simulink model "SiDLEngine"  (R2021b)
settings: Solver=VariableStepAuto  StartTime=0.0  StopTime=inf  FixedStep=0.03  RelTol=1e-3  EnableMultiTasking=on
model workspace (MAT data in the model file):
  AfrStoich = Simulink.Parameter
  AfrStoich.Value = 14.6
  AfrStoich.DataType = 'double'
  AfrStoich.Complexity = 'real'
  AfrStoich.Dimensions = [1 1]
  Cps = Simulink.Parameter
  Cps.Value = 2
  Cps.DataType = 'double'
  Cps.Complexity = 'real'
  Cps.Dimensions = [1 1]
  FuelSg = Simulink.Parameter
  FuelSg.Value = 0.75
  FuelSg.DataType = 'double'
  FuelSg.Complexity = 'real'
  FuelSg.Dimensions = [1 1]
  NCyl = Simulink.Parameter
  NCyl.Value = 4
  NCyl.DataType = 'double'
  NCyl.Complexity = 'real'
  NCyl.Dimensions = [1 1]
  Pstd = Simulink.Parameter
  Pstd.Value = 101325
  Pstd.DataType = 'double'
  Pstd.Complexity = 'real'
  Pstd.Dimensions = [1 1]
  Rair = Simulink.Parameter
  Rair.Value = 287
  Rair.DataType = 'double'
  Rair.Complexity = 'real'
  Rair.Dimensions = [1 1]
  TimeCnstECP = Simulink.Parameter
  TimeCnstECP.Value = 0.01
  TimeCnstECP.DataType = 'double'
  TimeCnstECP.Complexity = 'real'
  TimeCnstECP.Dimensions = [1 1]
  TimeCnstEGR = Simulink.Parameter
  TimeCnstEGR.Value = 0.01
  TimeCnstEGR.DataType = 'double'
  TimeCnstEGR.Complexity = 'real'
  TimeCnstEGR.Dimensions = [1 1]
  TimeCnstETC = Simulink.Parameter
  TimeCnstETC.Value = 0.01
  TimeCnstETC.DataType = 'double'
  TimeCnstETC.Complexity = 'real'
  TimeCnstETC.Dimensions = [1 1]
  TimeCnstICP = Simulink.Parameter
  TimeCnstICP.Value = 0.01
  TimeCnstICP.DataType = 'double'
  TimeCnstICP.Complexity = 'real'
  TimeCnstICP.Dimensions = [1 1]
  TimeCnstIVL = Simulink.Parameter
  TimeCnstIVL.Value = 0.125
  TimeCnstIVL.DataType = 'double'
  TimeCnstIVL.Complexity = 'real'
  TimeCnstIVL.Dimensions = [1 1]
  TimeCnstMFA = Simulink.Parameter
  TimeCnstMFA.Value = 0.125
  TimeCnstMFA.DataType = 'double'
  TimeCnstMFA.Complexity = 'real'
  TimeCnstMFA.Dimensions = [1 1]
  TimeCnstSWVA = Simulink.Parameter
  TimeCnstSWVA.Value = 0.125
  TimeCnstSWVA.DataType = 'double'
  TimeCnstSWVA.Complexity = 'real'
  TimeCnstSWVA.Dimensions = [1 1]
  TimeCnstVCR = Simulink.Parameter
  TimeCnstVCR.Value = 0.125
  TimeCnstVCR.DataType = 'double'
  TimeCnstVCR.Complexity = 'real'
  TimeCnstVCR.Dimensions = [1 1]
  TimeCnstVGT = Simulink.Parameter
  TimeCnstVGT.Value = 0.15
  TimeCnstVGT.DataType = 'double'
  TimeCnstVGT.Complexity = 'real'
  TimeCnstVGT.Dimensions = [1 1]
  TimeCnstVIRL = Simulink.Parameter
  TimeCnstVIRL.Value = 0.125
  TimeCnstVIRL.DataType = 'double'
  TimeCnstVIRL.Complexity = 'real'
  TimeCnstVIRL.Dimensions = [1 1]
  TimeCnstWGA = Simulink.Parameter
  TimeCnstWGA.Value = 0.01
  TimeCnstWGA.DataType = 'double'
  TimeCnstWGA.Complexity = 'real'
  TimeCnstWGA.Dimensions = [1 1]
  Ts = Simulink.Parameter
  Ts.Value = 0.01
  Ts.DataType = 'double'
  Ts.Complexity = 'real'
  Ts.Dimensions = [1 1]
  Tstd = Simulink.Parameter
  Tstd.Value = 293.15
  Tstd.DataType = 'double'
  Tstd.Complexity = 'real'
  Tstd.Dimensions = [1 1]
  Vd = Simulink.Parameter
  Vd.Value = 0.0015
  Vd.DataType = 'double'
  Vd.Complexity = 'real'
  Vd.Dimensions = [1 1]
  layer2Bias = Simulink.Parameter
  layer2Bias.Value = [-0.102818198502 -0.0669189542532 -0.0175336152315 -0.0613032355905 -0.0570961982012 -0.061625469476 -0.0630445405841 -0.102546460927 -0.0423759259284 -0.0306564457715 -0.0652378797531 -0.129787817597 ... (800 elements, 800x1)]
  layer2Bias.DataType = 'single'
  layer2Bias.Complexity = 'real'
  layer2Bias.Dimensions = [800 1]
  layer2InputWeights = Simulink.Parameter
  layer2InputWeights.Value = [-0.0867959260941 0.0265881456435 -0.00261938013136 0.0648385435343 -0.0334306880832 -0.044301789254 0.0604524612427 0.00893297791481 -0.0994751527905 0.0255589019507 -0.122370123863 -0.0740034654737 ... (1600 elements, 800x2)]
  layer2InputWeights.DataType = 'single'
  layer2InputWeights.Complexity = 'real'
  layer2InputWeights.Dimensions = [800 2]
  layer2RecurrentWeights = Simulink.Parameter
  layer2RecurrentWeights.Value = [-0.015235141851 -0.11403311789 0.112884886563 0.0588350631297 0.0682250186801 0.0444636531174 -0.0968889594078 -0.0397337339818 -0.0227067749947 0.0294026453048 -0.0304179247469 -0.145884677768 ... (160000 elements, 800x200)]
  layer2RecurrentWeights.DataType = 'single'
  layer2RecurrentWeights.Complexity = 'real'
  layer2RecurrentWeights.Dimensions = [800 200]
  layer3Bias = Simulink.Parameter
  layer3Bias.Value = [0.0529259070754; 0.0636636316776; 0.0140457563102; 0.0780845806003; 0.0347621031106; -0.023198319599; -0.0368600413203; -0.00711429771036; -0.0257519558072; 0.0254531633109; 0.0144603000954]
  layer3Bias.DataType = 'single'
  layer3Bias.Complexity = 'real'
  layer3Bias.Dimensions = [11 1]
  layer3Weights = Simulink.Parameter
  layer3Weights.Value = [0.0566984564066 0.0242331400514 0.158808469772 0.0399505831301 -0.0030719502829 0.0837587192655 0.0579013302922 -0.0333247296512 -0.120384372771 -0.125806882977 0.0938690528274 -0.052338026464 ... (2200 elements, 11x200)]
  layer3Weights.DataType = 'single'
  layer3Weights.Complexity = 'real'
  layer3Weights.Dimensions = [11 200]
  muX = Simulink.Parameter
  muX.Value = [2220.83734119 107.92815484]
  muX.DataType = 'double'
  muX.Complexity = 'real'
  muX.Dimensions = [1 2]
  muY = Simulink.Parameter
  muY.Value = [104.671657967 115562.072489 0.00224719893222 986.056400633 7383.06398882 0.0299760704621 325.741103054 5.88867806863e-05 0.000942478781448 3.56158507349e-05 0.00543639293543]
  muY.DataType = 'double'
  muY.Complexity = 'real'
  muY.Dimensions = [1 11]
  sigX = Simulink.Parameter
  sigX.Value = [1470.27383875 63.5647381428]
  sigX.DataType = 'double'
  sigX.Complexity = 'real'
  sigX.Dimensions = [1 2]
  sigY = Simulink.Parameter
  sigY.Value = [65.6275263528 46686.4071583 0.00207427504126 224.539922164 5111.0011239 0.0252132241042 8.06209455442 0.000125926264941 0.00171123843744 4.89959895827e-05 0.00480295587248]
  sigY.DataType = 'double'
  sigY.Complexity = 'real'
  sigY.Dimensions = [1 11]
libraries: autolibutils x4, simulink x2, autolibsharedmappedenginescommon x1, autolibpowerinfoutils x1
settings Model: DataDictionary=SiDLEngine.sldd  ModifiedByFormat=The MathWorks, Inc.  Creator=The MathWorks, Inc.  LastModifiedBy=The MathWorks, Inc.
settings SolverCC: AlgebraicLoopSolver=TrustRegion  DecoupledContinuousIntegration=on
settings DataIOCC: DSMLogging=off  ReturnWorkspaceOutputs=off
settings DebuggingCC: SFMachineParentedDataDiag=warning  ArithmeticOperatorsInVariantConditions=warning
settings SFSimCC: SimUseLocalCustomCode=off
settings RTWCC: RTWUseLocalCustomCode=off
settings CodeAppCC: StateflowObjectComments=on
settings GRTTargetCC: TargetLangStandard=C89/C90 (ANSI)
settings ConfigComp: CovMetricSettings=dsw  CovSaveCumulativeToWorkspaceVar=on  CovSaveSingleToWorkspaceVar=on  CovExternalEMLEnable=off
settings SimscapeCC: SimscapeNormalizeSystem=off  SimscapeNominalValues={1, 'bar'; 1, 'cm^3/s'; 1, 'bar*kg/s'; 1, 'kJ/kg'; 1, 'kW'}

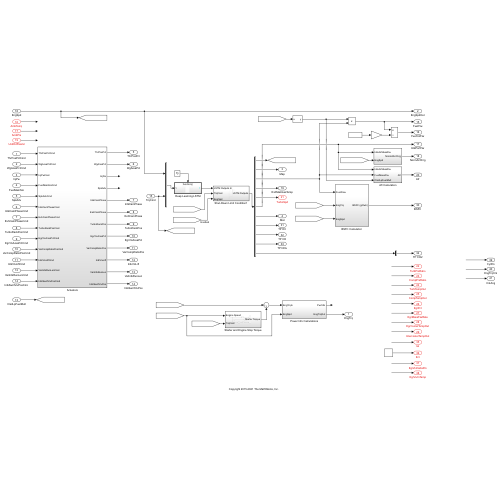
[thumbnail: Simulink's stored preview of the top-level diagram]
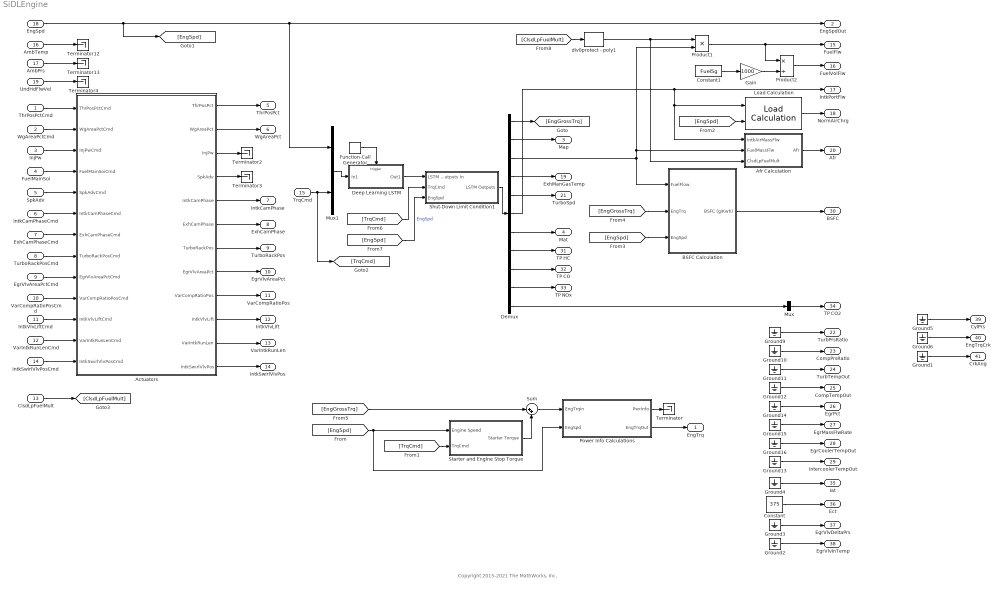
== system SiDLEngine ==
  note: Copyright 2015-2021 The MathWorks, Inc.
  ThrPosPctCmd : Inport
  WgAreaPctCmd : Inport  Port=2
  InjPw : Inport  Port=3
  FuelMainSoi : Inport  Port=4
  SpkAdv : Inport  Port=5
  IntkCamPhaseCmd : Inport  Port=6
  ExhCamPhaseCmd : Inport  Port=7
  TurboRackPosCmd : Inport  Port=8
  EgrVlvAreaPctCmd : Inport  Port=9
  VarCompRatioPosCmd : Inport  Port=10
  IntkVlvLiftCmd : Inport  Port=11
  VarIntkRunLenCmd : Inport  Port=12
  ClsdLpFuelMult : Inport  Port=13  Unit=1
  IntkSwirlVlvPosCmd : Inport  Port=14
  TrqCmd : Inport  Port=15  Unit=N*m
  AmbTemp : Inport  Port=16  Unit=K
  AmbPrs : Inport  Port=17  Unit=Pa
  EngSpd : Inport  Port=18  Interpolate=off
  UndHdFlwVel : Inport  Port=19  Unit=m/s
  Actuators : Subsystem
  Afr Calculation : Subsystem
  BSFC Calculation : Subsystem
  Constant : Constant  Value=375
  Constant1 : Constant  Value=FuelSg
  Deep Learning LSTM : Subsystem  TreatAsAtomicUnit=on
  Demux : Demux  Outputs=11
  Function-Call Generator : simulink/Ports & Subsystems/Function-Call Generator  sample_time=Ts  numberOfIterations=1  DisallowWideOutput=off
  Gain : Gain  Gain=1000
  Ground{1..6,9..16} (14 alike) : Ground
  Load Calculation : autolibsharedmappedenginescommon/Load Calculation  SystemSampleTime=-1  VariantActivationTime=update diagram  Latency=0  AutoFrameSizeCalculation=off
      settings: SourceProductBaseCode=PW,DR,MT,UV,VE
  Mux : Mux  Inputs=1
  Mux1 : Mux  Inputs=2
  Power Info Calculations : Subsystem
  Product1 : Product
  Product2 : Product  Inputs=*/
  Shut-Down Limit Condition1 : Subsystem
  Starter and Engine Stop Torque : Subsystem
  Sum : Sum  Inputs=|++
  Terminator{,2..4,12..13} (6 alike) : Terminator
  div0protect - poly1 : autolibutils/div0protect - poly  thresh=0.01  ZeroCross1=off  aMode=aMode
      settings: SourceProductBaseCode=PW,DR,MT,UV,VE
  EngTrq : Outport  Unit=N*m  VectorParamsAs1DForOutWhenUnconnected=off
  EngSpdOut : Outport  Port=2  VectorParamsAs1DForOutWhenUnconnected=off
  Map : Outport  Port=3  Unit=Pa  VectorParamsAs1DForOutWhenUnconnected=off
  Mat : Outport  Port=4  Unit=K  VectorParamsAs1DForOutWhenUnconnected=off
  ThrPosPct : Outport  Port=5  VectorParamsAs1DForOutWhenUnconnected=off
  WgAreaPct : Outport  Port=6  VectorParamsAs1DForOutWhenUnconnected=off
  IntkCamPhase : Outport  Port=7  VectorParamsAs1DForOutWhenUnconnected=off
  ExhCamPhase : Outport  Port=8  VectorParamsAs1DForOutWhenUnconnected=off
  TurboRackPos : Outport  Port=9  VectorParamsAs1DForOutWhenUnconnected=off
  EgrVlvAreaPct : Outport  Port=10  VectorParamsAs1DForOutWhenUnconnected=off
  VarCompRatioPos : Outport  Port=11  VectorParamsAs1DForOutWhenUnconnected=off
  IntkVlvLift : Outport  Port=12  VectorParamsAs1DForOutWhenUnconnected=off
  VarIntkRunLen : Outport  Port=13  VectorParamsAs1DForOutWhenUnconnected=off
  IntkSwirlVlvPos : Outport  Port=14  VectorParamsAs1DForOutWhenUnconnected=off
  FuelFlw : Outport  Port=15  Unit=kg/s  VectorParamsAs1DForOutWhenUnconnected=off
  FuelVolFlw : Outport  Port=16  Unit=m^3/s  VectorParamsAs1DForOutWhenUnconnected=off
  IntkPortFlw : Outport  Port=17  Unit=kg/s  VectorParamsAs1DForOutWhenUnconnected=off
  NormAirChrg : Outport  Port=18  Unit=1  VectorParamsAs1DForOutWhenUnconnected=off
  ExhManGasTemp : Outport  Port=19  Unit=K  VectorParamsAs1DForOutWhenUnconnected=off
  Afr : Outport  Port=20  Unit=1  VectorParamsAs1DForOutWhenUnconnected=off
  TurboSpd : Outport  Port=21  Unit=rad/s  VectorParamsAs1DForOutWhenUnconnected=off
  TurbPrsRatio : Outport  Port=22  Unit=1  VectorParamsAs1DForOutWhenUnconnected=off
  CompPrsRatio : Outport  Port=23  Unit=1  VectorParamsAs1DForOutWhenUnconnected=off
  TurbTempOut : Outport  Port=24  Unit=K  VectorParamsAs1DForOutWhenUnconnected=off
  CompTempOut : Outport  Port=25  Unit=K  VectorParamsAs1DForOutWhenUnconnected=off
  EgrPct : Outport  Port=26  Unit=%  VectorParamsAs1DForOutWhenUnconnected=off
  EgrMassFlwRate : Outport  Port=27  Unit=kg/s  VectorParamsAs1DForOutWhenUnconnected=off
  EgrCoolerTempOut : Outport  Port=28  Unit=K  VectorParamsAs1DForOutWhenUnconnected=off
  IntercoolerTempOut : Outport  Port=29  Unit=K  VectorParamsAs1DForOutWhenUnconnected=off
  BSFC : Outport  Port=30  Unit=g/(kW*hr)  VectorParamsAs1DForOutWhenUnconnected=off
  TP HC : Outport  Port=31  Unit=kg/s  VectorParamsAs1DForOutWhenUnconnected=off
  TP CO : Outport  Port=32  Unit=kg/s  VectorParamsAs1DForOutWhenUnconnected=off
  TP NOx : Outport  Port=33  Unit=kg/s  VectorParamsAs1DForOutWhenUnconnected=off
  TP CO2 : Outport  Port=34  Unit=kg/s  VectorParamsAs1DForOutWhenUnconnected=off
  Iat : Outport  Port=35  Unit=K  VectorParamsAs1DForOutWhenUnconnected=off
  Ect : Outport  Port=36  Unit=K  VectorParamsAs1DForOutWhenUnconnected=off
  EgrVlvDeltaPrs : Outport  Port=37  Unit=Pa  VectorParamsAs1DForOutWhenUnconnected=off
  EgrVlvInTemp : Outport  Port=38  Unit=K  VectorParamsAs1DForOutWhenUnconnected=off
  CylPrs : Outport  Port=39  VectorParamsAs1DForOutWhenUnconnected=off
  EngTrqCrk : Outport  Port=40  VectorParamsAs1DForOutWhenUnconnected=off
  CrkAng : Outport  Port=41  VectorParamsAs1DForOutWhenUnconnected=off
  wires:
  Demux/6 -> Load Calculation/1, Afr Calculation/1(IntkAirMassFlw), IntkPortFlw/1
  Demux/11 -> Mux/1
  Demux/9 -> TP CO/1
  Mux/1 -> TP CO2/1
  IntkCamPhaseCmd/1 -> Actuators/6(IntkCamPhaseCmd)
  Ground16/1 -> EgrCoolerTempOut/1
  Ground13/1 -> IntercoolerTempOut/1
  Ground12/1 -> CompTempOut/1
  FuelMainSoi/1 -> Actuators/4(FuelMainSoiCmd)
  EgrVlvAreaPctCmd/1 -> Actuators/9(EgrVlvAreaPctCmd)
  Ground11/1 -> TurbTempOut/1
  ExhCamPhaseCmd/1 -> Actuators/7(ExhCamPhaseCmd)
  Ground9/1 -> TurbPrsRatio/1
  SpkAdv/1 -> Actuators/5(SpkAdvCmd)
  AmbTemp/1 -> Terminator12/1
  Ground15/1 -> EgrMassFlwRate/1
  TurboRackPosCmd/1 -> Actuators/8(TurboRackPosCmd)
  ThrPosPctCmd/1 -> Actuators/1(ThrPosPctCmd)
  WgAreaPctCmd/1 -> Actuators/2(WgAreaPctCmd)
  InjPw/1 -> Actuators/3(InjPwCmd)
  Ground10/1 -> CompPrsRatio/1
  Demux/7 -> Mat/1
  Demux/2 -> Map/1
  AmbPrs/1 -> Terminator13/1
  IntkVlvLiftCmd/1 -> Actuators/11(IntkVlvLiftCmd)
  VarCompRatioPosCmd/1 -> Actuators/10(VarCompRatioPosCmd)
  VarIntkRunLenCmd/1 -> Actuators/12(VarIntkRunLenCmd)
  IntkSwirlVlvPosCmd/1 -> Actuators/13(IntkSwirlVlvPosCmd)
  UndHdFlwVel/1 -> Terminator4/1
  Actuators/5(IntkCamPhase) -> IntkCamPhase/1
  Actuators/6(ExhCamPhase) -> ExhCamPhase/1
  Actuators/7(TurboRackPos) -> TurboRackPos/1
  Actuators/8(EgrVlvAreaPct) -> EgrVlvAreaPct/1
  Actuators/9(VarCompRatioPos) -> VarCompRatioPos/1
  Actuators/10(IntkVlvLift) -> IntkVlvLift/1
  Actuators/11(VarIntkRunLen) -> VarIntkRunLen/1
  Actuators/12(IntkSwirlVlvPos) -> IntkSwirlVlvPos/1
  Constant/1 -> Ect/1
  Ground2/1 -> EgrVlvInTemp/1
  Ground3/1 -> EgrVlvDeltaPrs/1
  Ground4/1 -> Iat/1
  Power Info Calculations/1(PwrInfo) -> Terminator/1
  Demux/3 -> Afr Calculation/2(FuelMassFlw), Product1/2, BSFC Calculation/1(FuelFlow)
  Product2/1 -> FuelVolFlw/1
  ClsdLpFuelMult/1 -> [ClsdLpFuelMult]
  Deep Learning LSTM/1(Out1) -> Shut-Down Limit Condition1/1(LSTM Outputs In)
  Demux/4 -> ExhManGasTemp/1
  Demux/5 -> TurboSpd/1
  Constant1/1 -> Gain/1
  Starter and Engine Stop Torque/1(Starter Torque) -> Sum/2
  Sum/1 -> Power Info Calculations/1(EngTrqIn)
  Function-Call Generator/1 -> Deep Learning LSTM/Trigger
  Ground14/1 -> EgrPct/1
  Gain/1 -> Product2/2
  Power Info Calculations/2(EngTrqOut) -> EngTrq/1
  [EngSpd] -> Starter and Engine Stop Torque/1(Engine Speed), Power Info Calculations/2(EngSpd)
  Afr Calculation/1(Afr) -> Afr/1
  Load Calculation/1 -> NormAirChrg/1
  [EngSpd] -> Load Calculation/2
  BSFC Calculation/1(BSFC (g/Kwh)) -> BSFC/1
  [EngSpd] -> BSFC Calculation/3(EngSpd)
  [EngGrossTrq] -> BSFC Calculation/2(EngTrq)
  [TrqCmd] -> Starter and Engine Stop Torque/2(TrqCmd)
  Shut-Down Limit Condition1/1(LSTM Outputs) -> Demux/1
  [EngSpd] -> Shut-Down Limit Condition1/3(EngSpd)  "EngSpd"
  EngSpd/1 -> [EngSpd], Mux1/1, EngSpdOut/1
  Actuators/1(ThrPosPct) -> ThrPosPct/1
  Actuators/2(WgAreaPct) -> WgAreaPct/1
  Actuators/3(InjPw) -> Terminator2/1
  Actuators/4(SpkAdv) -> Terminator3/1
  [EngGrossTrq] -> Sum/1
  Mux1/1 -> Deep Learning LSTM/1(In1)
  Demux/1 -> [EngGrossTrq]
  TrqCmd/1 -> [TrqCmd], Mux1/2
  Demux/8 -> TP HC/1
  Demux/10 -> TP NOx/1
  [TrqCmd] -> Shut-Down Limit Condition1/2(TrqCmd)
  [ClsdLpFuelMult] -> div0protect - poly1/1
  Product1/1 -> Product2/1, FuelFlw/1
  div0protect - poly1/1 -> Afr Calculation/3(ClsdLpFuelMult), Product1/1
  Ground5/1 -> CylPrs/1
  Ground6/1 -> EngTrqCrk/1
  Ground1/1 -> CrkAng/1

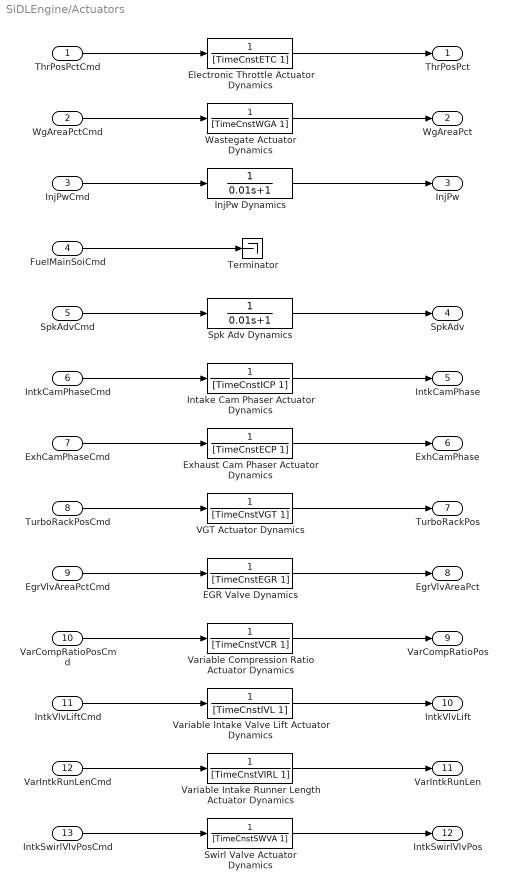
== system SiDLEngine/Actuators ==
  ThrPosPctCmd : Inport  Unit=%
  WgAreaPctCmd : Inport  Port=2  Unit=%
  InjPwCmd : Inport  Port=3  Unit=ms
  FuelMainSoiCmd : Inport  Port=4  Unit=deg
  SpkAdvCmd : Inport  Port=5  Unit=deg
  IntkCamPhaseCmd : Inport  Port=6  Unit=deg
  ExhCamPhaseCmd : Inport  Port=7  Unit=deg
  TurboRackPosCmd : Inport  Port=8  Unit=1
  EgrVlvAreaPctCmd : Inport  Port=9  Unit=%
  VarCompRatioPosCmd : Inport  Port=10
  IntkVlvLiftCmd : Inport  Port=11
  VarIntkRunLenCmd : Inport  Port=12
  IntkSwirlVlvPosCmd : Inport  Port=13
  EGR Valve Dynamics : TransferFcn  Denominator=[TimeCnstEGR 1]
  Electronic Throttle Actuator Dynamics : TransferFcn  Denominator=[TimeCnstETC 1]
  Exhaust Cam Phaser Actuator Dynamics : TransferFcn  Denominator=[TimeCnstECP 1]
  InjPw Dynamics : TransferFcn  Denominator=[0.01 1]
  Intake Cam Phaser Actuator Dynamics : TransferFcn  Denominator=[TimeCnstICP 1]
  Spk Adv Dynamics : TransferFcn  Denominator=[0.01 1]
  Swirl Valve Actuator Dynamics : TransferFcn  Denominator=[TimeCnstSWVA 1]
  Terminator : Terminator
  VGT Actuator Dynamics : TransferFcn  Denominator=[TimeCnstVGT 1]
  Variable Compression Ratio Actuator Dynamics : TransferFcn  Denominator=[TimeCnstVCR 1]
  Variable Intake Runner Length Actuator Dynamics : TransferFcn  Denominator=[TimeCnstVIRL 1]
  Variable Intake Valve Lift Actuator Dynamics : TransferFcn  Denominator=[TimeCnstIVL 1]
  Wastegate Actuator Dynamics : TransferFcn  Denominator=[TimeCnstWGA 1]
  ThrPosPct : Outport  Unit=%  VectorParamsAs1DForOutWhenUnconnected=off
  WgAreaPct : Outport  Port=2  Unit=%  VectorParamsAs1DForOutWhenUnconnected=off
  InjPw : Outport  Port=3  VectorParamsAs1DForOutWhenUnconnected=off
  SpkAdv : Outport  Port=4  VectorParamsAs1DForOutWhenUnconnected=off
  IntkCamPhase : Outport  Port=5  Unit=deg  VectorParamsAs1DForOutWhenUnconnected=off
  ExhCamPhase : Outport  Port=6  Unit=deg  VectorParamsAs1DForOutWhenUnconnected=off
  TurboRackPos : Outport  Port=7  Unit=1  VectorParamsAs1DForOutWhenUnconnected=off
  EgrVlvAreaPct : Outport  Port=8  Unit=%  VectorParamsAs1DForOutWhenUnconnected=off
  VarCompRatioPos : Outport  Port=9  VectorParamsAs1DForOutWhenUnconnected=off
  IntkVlvLift : Outport  Port=10  VectorParamsAs1DForOutWhenUnconnected=off
  VarIntkRunLen : Outport  Port=11  VectorParamsAs1DForOutWhenUnconnected=off
  IntkSwirlVlvPos : Outport  Port=12  VectorParamsAs1DForOutWhenUnconnected=off
  wires:
  Variable Compression Ratio Actuator Dynamics/1 -> VarCompRatioPos/1
  Variable Intake Valve Lift Actuator Dynamics/1 -> IntkVlvLift/1
  Variable Intake Runner Length Actuator Dynamics/1 -> VarIntkRunLen/1
  Swirl Valve Actuator Dynamics/1 -> IntkSwirlVlvPos/1
  Intake Cam Phaser Actuator Dynamics/1 -> IntkCamPhase/1
  Exhaust Cam Phaser Actuator Dynamics/1 -> ExhCamPhase/1
  Wastegate Actuator Dynamics/1 -> WgAreaPct/1
  Electronic Throttle Actuator Dynamics/1 -> ThrPosPct/1
  FuelMainSoiCmd/1 -> Terminator/1
  IntkVlvLiftCmd/1 -> Variable Intake Valve Lift Actuator Dynamics/1
  IntkSwirlVlvPosCmd/1 -> Swirl Valve Actuator Dynamics/1
  WgAreaPctCmd/1 -> Wastegate Actuator Dynamics/1
  ThrPosPctCmd/1 -> Electronic Throttle Actuator Dynamics/1
  ExhCamPhaseCmd/1 -> Exhaust Cam Phaser Actuator Dynamics/1
  IntkCamPhaseCmd/1 -> Intake Cam Phaser Actuator Dynamics/1
  VarCompRatioPosCmd/1 -> Variable Compression Ratio Actuator Dynamics/1
  VarIntkRunLenCmd/1 -> Variable Intake Runner Length Actuator Dynamics/1
  InjPwCmd/1 -> InjPw Dynamics/1
  VGT Actuator Dynamics/1 -> TurboRackPos/1
  EGR Valve Dynamics/1 -> EgrVlvAreaPct/1
  TurboRackPosCmd/1 -> VGT Actuator Dynamics/1
  EgrVlvAreaPctCmd/1 -> EGR Valve Dynamics/1
  SpkAdvCmd/1 -> Spk Adv Dynamics/1
  Spk Adv Dynamics/1 -> SpkAdv/1
  InjPw Dynamics/1 -> InjPw/1

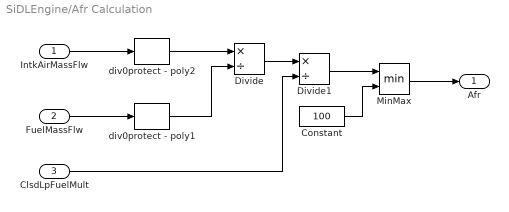
== system SiDLEngine/Afr Calculation ==
  IntkAirMassFlw : Inport  Unit=kg/s
  FuelMassFlw : Inport  Port=2  Unit=kg/s
  ClsdLpFuelMult : Inport  Port=3  Unit=kg/s
  Constant : Constant  Value=100
  Divide : Product  Inputs=*/
  Divide1 : Product  Inputs=*/
  MinMax : MinMax  Inputs=2  ZeroCross=off
  div0protect - poly1 : autolibutils/div0protect - poly  thresh=1e-9  ZeroCross1=off  aMode=aMode
      settings: SourceProductBaseCode=PW,DR,MT,UV,VE
  div0protect - poly2 : autolibutils/div0protect - poly  thresh=100e-9  ZeroCross1=off  aMode=aMode
      settings: SourceProductBaseCode=PW,DR,MT,UV,VE
  Afr : Outport  Unit=1  VectorParamsAs1DForOutWhenUnconnected=off
  wires:
  MinMax/1 -> Afr/1
  div0protect - poly1/1 -> Divide/2
  Divide/1 -> Divide1/1
  div0protect - poly2/1 -> Divide/1
  Constant/1 -> MinMax/2
  IntkAirMassFlw/1 -> div0protect - poly2/1
  FuelMassFlw/1 -> div0protect - poly1/1
  ClsdLpFuelMult/1 -> Divide1/2
  Divide1/1 -> MinMax/1

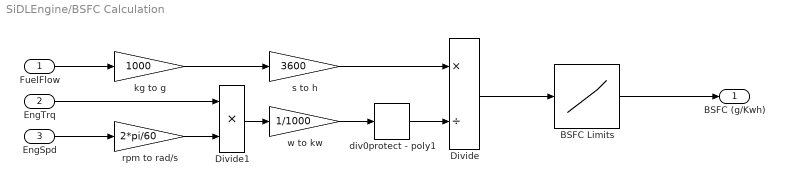
== system SiDLEngine/BSFC Calculation ==
  FuelFlow : Inport
  EngTrq : Inport  Port=2
  EngSpd : Inport  Port=3
  BSFC Limits : Lookup_n-D  NumberOfTableDimensions=1  BreakpointsForDimension1=[0 500]  Table=[0 500]  ExtrapMethod=Clip  InternalRulePriority=Speed  RndMeth=Simplest  InputSameDT=on
  Divide : Product  Inputs=*/
  Divide1 : Product  Inputs=**
  div0protect - poly1 : autolibutils/div0protect - poly  thresh=1e-6  ZeroCross1=off  aMode=aMode
      settings: SourceProductBaseCode=PW,DR,MT,UV,VE
  kg to g : Gain  Gain=1000
  rpm to rad/s : Gain  Gain=2*pi/60
  s to h : Gain  Gain=3600
  w to kw : Gain  Gain=1/1000
  BSFC (g/Kwh) : Outport  VectorParamsAs1DForOutWhenUnconnected=off
  wires:
  Divide1/1 -> w to kw/1
  kg to g/1 -> s to h/1
  FuelFlow/1 -> kg to g/1
  rpm to rad/s/1 -> Divide1/2
  EngSpd/1 -> rpm to rad/s/1
  EngTrq/1 -> Divide1/1
  Divide/1 -> BSFC Limits/1
  w to kw/1 -> div0protect - poly1/1
  s to h/1 -> Divide/1
  BSFC Limits/1 -> BSFC (g/Kwh)/1
  div0protect - poly1/1 -> Divide/2

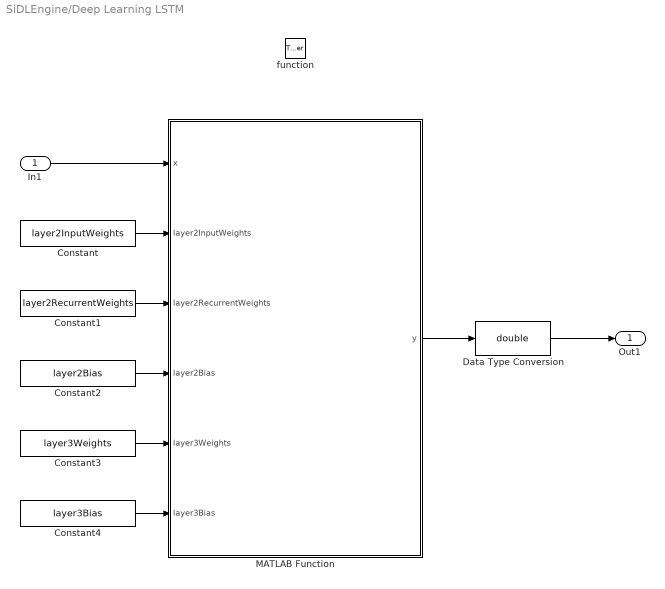
== system SiDLEngine/Deep Learning LSTM ==
  In1 : Inport
  function : TriggerPort  TriggerType=function-call  VariantControl=Variant
  Constant : Constant  Value=layer2InputWeights
  Constant1 : Constant  Value=layer2RecurrentWeights
  Constant2 : Constant  Value=layer2Bias
  Constant3 : Constant  Value=layer3Weights
  Constant4 : Constant  Value=layer3Bias
  Data Type Conversion : DataTypeConversion  OutDataTypeStr=double
  MATLAB Function : MATLAB Function  TreatAsAtomicUnit=on
  Out1 : Outport  VectorParamsAs1DForOutWhenUnconnected=off
  wires:
  In1/1 -> MATLAB Function/1(x)
  MATLAB Function/1(y) -> Data Type Conversion/1
  Data Type Conversion/1 -> Out1/1
  Constant/1 -> MATLAB Function/2(layer2InputWeights)
  Constant1/1 -> MATLAB Function/3(layer2RecurrentWeights)
  Constant2/1 -> MATLAB Function/4(layer2Bias)
  Constant3/1 -> MATLAB Function/5(layer3Weights)
  Constant4/1 -> MATLAB Function/6(layer3Bias)

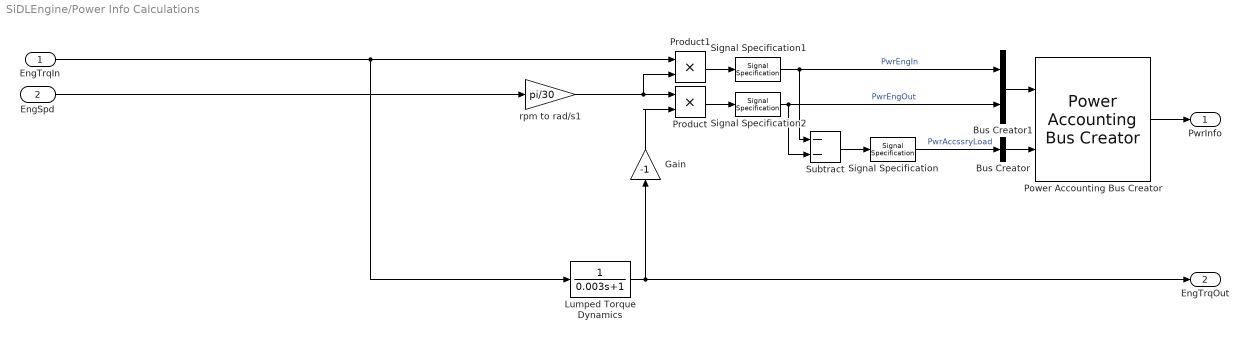
== system SiDLEngine/Power Info Calculations ==
  EngTrqIn : Inport
  EngSpd : Inport  Port=2
  Bus Creator : BusCreator  Inputs=1
  Bus Creator1 : BusCreator  Inputs=2
  Gain : Gain  Gain=-1
  Lumped Torque Dynamics : TransferFcn  Denominator=[0.003 1]
  Power Accounting Bus Creator : autolibpowerinfoutils/Power Accounting Bus Creator  AssctBlkSelPopup=Parent  RefBlkName='libraryname/blkname'  PwrTrnsfrdCheckBox=on  PwrNotTrnsfrdCheckBox=on  PwrStoredCheckBox=off  aMode=aMode
      settings: SourceProductBaseCode=PW,DR,MT,UV,VE
  Product : Product
  Product1 : Product
  Signal Specification : SignalSpecification  Unit=W
  Signal Specification1 : SignalSpecification  Unit=W
  Signal Specification2 : SignalSpecification  Unit=W
  Subtract : Sum  Inputs=--
  rpm to rad/s1 : Gain  Gain=pi/30
  PwrInfo : Outport  VectorParamsAs1DForOutWhenUnconnected=off
  EngTrqOut : Outport  Port=2  Unit=N*m  VectorParamsAs1DForOutWhenUnconnected=off
  wires:
  EngSpd/1 -> rpm to rad/s1/1
  Lumped Torque Dynamics/1 -> EngTrqOut/1, Gain/1
  Bus Creator/1 -> Power Accounting Bus Creator/2
  Bus Creator1/1 -> Power Accounting Bus Creator/1
  EngTrqIn/1 -> Lumped Torque Dynamics/1, Product1/1
  Subtract/1 -> Signal Specification/1
  Signal Specification/1 -> Bus Creator/1  "PwrAccssryLoad"
  Power Accounting Bus Creator/1 -> PwrInfo/1
  Product/1 -> Signal Specification2/1
  Product1/1 -> Signal Specification1/1
  rpm to rad/s1/1 -> Product1/2, Product/1
  Signal Specification1/1 -> Subtract/1, Bus Creator1/1  "PwrEngIn"
  Signal Specification2/1 -> Subtract/2, Bus Creator1/2  "PwrEngOut"
  Gain/1 -> Product/2

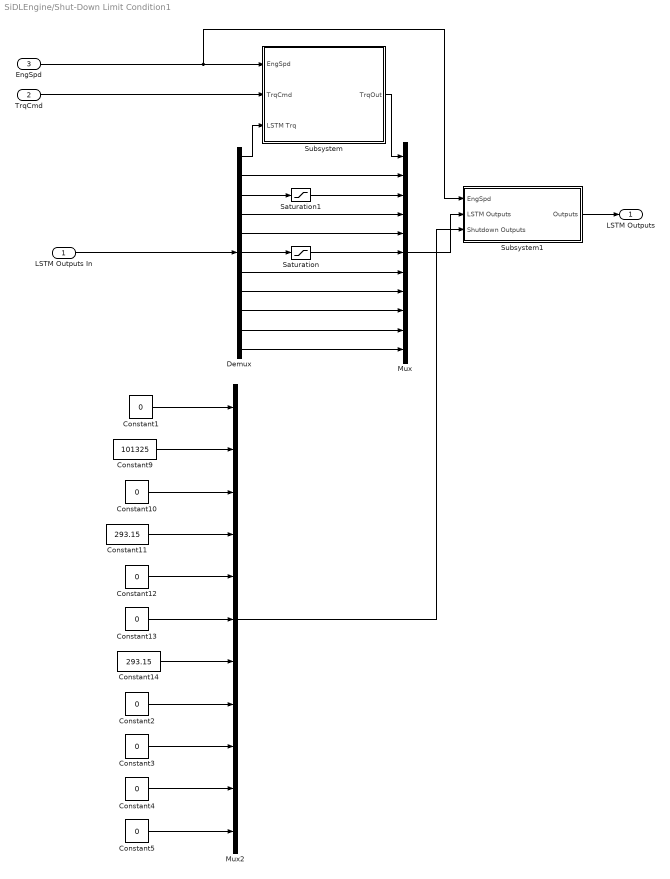
== system SiDLEngine/Shut-Down Limit Condition1 ==
  LSTM Outputs In : Inport
  TrqCmd : Inport  Port=2
  EngSpd : Inport  Port=3
  Constant{1..5,10,12..13} (8 alike) : Constant  Value=0
  Constant11 : Constant  Value=293.15
  Constant14 : Constant  Value=293.15
  Constant9 : Constant  Value=101325
  Demux : Demux  Outputs=11
  Mux : Mux  Inputs=11
  Mux2 : Mux  Inputs=11
  Saturation : Saturate  UpperLimit=inf  LowerLimit=0
  Saturation1 : Saturate  UpperLimit=inf  LowerLimit=0
  Subsystem : Subsystem
  Subsystem1 : Subsystem
  LSTM Outputs : Outport  VectorParamsAs1DForOutWhenUnconnected=off
  wires:
  EngSpd/1 -> Subsystem1/1(EngSpd), Subsystem/1(EngSpd)
  LSTM Outputs In/1 -> Demux/1
  Demux/7 -> Mux/7
  Demux/6 -> Saturation/1
  Demux/5 -> Mux/5
  Demux/4 -> Mux/4
  Demux/3 -> Saturation1/1
  Demux/2 -> Mux/2
  Demux/1 -> Subsystem/3(LSTM Trq)
  Subsystem/1(TrqOut) -> Mux/1
  Subsystem1/1(Outputs) -> LSTM Outputs/1
  Mux/1 -> Subsystem1/2(LSTM Outputs)
  TrqCmd/1 -> Subsystem/2(TrqCmd)
  Constant2/1 -> Mux2/8
  Mux2/1 -> Subsystem1/3(Shutdown Outputs)
  Constant5/1 -> Mux2/11
  Constant3/1 -> Mux2/9
  Constant4/1 -> Mux2/10
  Constant12/1 -> Mux2/5
  Constant1/1 -> Mux2/1
  Constant10/1 -> Mux2/3
  Constant9/1 -> Mux2/2
  Constant13/1 -> Mux2/6
  Constant14/1 -> Mux2/7
  Constant11/1 -> Mux2/4
  Demux/8 -> Mux/8
  Demux/9 -> Mux/9
  Demux/10 -> Mux/10
  Demux/11 -> Mux/11
  Saturation/1 -> Mux/6
  Saturation1/1 -> Mux/3

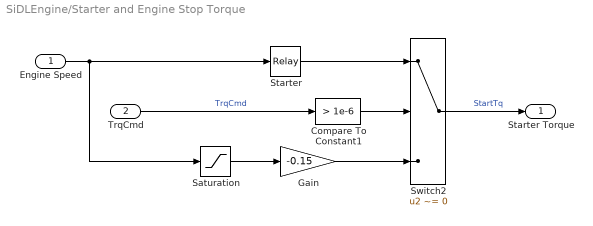
== system SiDLEngine/Starter and Engine Stop Torque ==
  Engine Speed : Inport
  TrqCmd : Inport  Port=2
  Compare To Constant1 : simulink/Logic and Bit Operations/Compare To Constant  relop=>  const=1e-6  OutDataTypeStr=boolean
  Gain : Gain  Gain=-0.15
  Saturation : Saturate  UpperLimit=100  LowerLimit=-100
  Starter : Relay  OnSwitchValue=300  OffSwitchValue=150  OnOutputValue=0  OffOutputValue=20
  Switch2 : Switch  Criteria=u2 ~= 0
  Starter Torque : Outport  VectorParamsAs1DForOutWhenUnconnected=off
  wires:
  Saturation/1 -> Gain/1
  Starter/1 -> Switch2/1
  TrqCmd/1 -> Compare To Constant1/1  "TrqCmd"
  Switch2/1 -> Starter Torque/1  "StartTq"
  Engine Speed/1 -> Starter/1, Saturation/1
  Compare To Constant1/1 -> Switch2/2
  Gain/1 -> Switch2/3

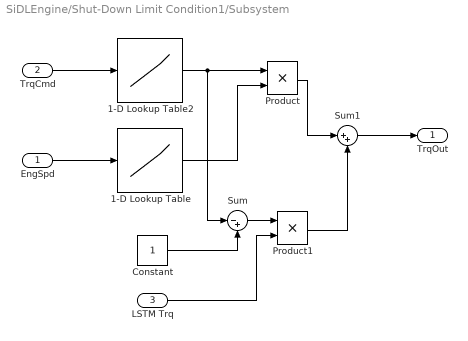
== system SiDLEngine/Shut-Down Limit Condition1/Subsystem ==
  EngSpd : Inport
  TrqCmd : Inport  Port=2
  LSTM Trq : Inport  Port=3
  1-D Lookup Table : Lookup_n-D  NumberOfTableDimensions=1  BreakpointsForDimension1="[0\t750\t1053.57142857143\t1357.14285714286\t1660.71428571429\t1964.28571428571\t2267.85714285714\t2571.42857142857\t2875\t3178.57142857143\t3482.14285714286\t3785.71428571429\t4089.28571428571\t4392.85714285714\t4696.42857142857\t5000]"  Table="[0\t-9.29036880275297\t-10.6228292739026\t-11.9924964963700\t-13.0118311605534\t-14.0012727910098\t-14.7810585236861\t-15.7592347457006\t-16.5866921936305\t-17.2855138761427\t-18.0323141674096\t-18.7301010682725\t-19.4167284926662\t-20.1293721332724\t-20.8757603607253\t-21.6717938972620]"  ExtrapMethod=Clip  InternalRulePriority=Speed  RndMeth=Simplest  InputSameDT=on
  1-D Lookup Table2 : Lookup_n-D  NumberOfTableDimensions=1  BreakpointsForDimension1=[0 1]*1e-6  Table=[1 0]  ExtrapMethod=Clip  InternalRulePriority=Speed  RndMeth=Simplest  InputSameDT=on
  Constant : Constant
  Product : Product
  Product1 : Product
  Sum : Sum  Inputs=|-+
  Sum1 : Sum  Inputs=|++
  TrqOut : Outport  VectorParamsAs1DForOutWhenUnconnected=off
  wires:
  EngSpd/1 -> 1-D Lookup Table/1
  Product/1 -> Sum1/1
  Sum/1 -> Product1/1
  1-D Lookup Table2/1 -> Product/1, Sum/1
  Constant/1 -> Sum/2
  Product1/1 -> Sum1/2
  1-D Lookup Table/1 -> Product/2
  TrqCmd/1 -> 1-D Lookup Table2/1
  Sum1/1 -> TrqOut/1
  LSTM Trq/1 -> Product1/2

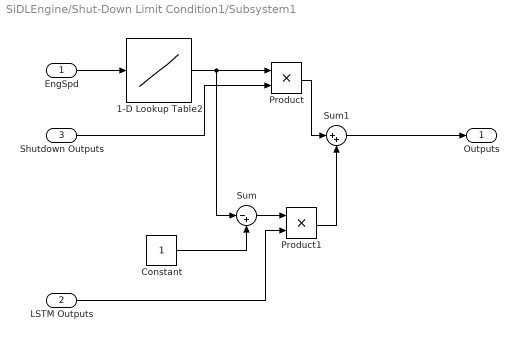
== system SiDLEngine/Shut-Down Limit Condition1/Subsystem1 ==
  EngSpd : Inport
  LSTM Outputs : Inport  Port=2
  Shutdown Outputs : Inport  Port=3
  1-D Lookup Table2 : Lookup_n-D  NumberOfTableDimensions=1  BreakpointsForDimension1=[0 1]  Table=[1 0]  ExtrapMethod=Clip  InternalRulePriority=Speed  RndMeth=Simplest  InputSameDT=on
  Constant : Constant
  Product : Product
  Product1 : Product
  Sum : Sum  Inputs=|-+
  Sum1 : Sum  Inputs=|++
  Outputs : Outport  VectorParamsAs1DForOutWhenUnconnected=off
  wires:
  Product/1 -> Sum1/1
  Sum/1 -> Product1/1
  1-D Lookup Table2/1 -> Sum/1, Product/1
  Constant/1 -> Sum/2
  Product1/1 -> Sum1/2
  Shutdown Outputs/1 -> Product/2
  Sum1/1 -> Outputs/1
  LSTM Outputs/1 -> Product1/2
  EngSpd/1 -> 1-D Lookup Table2/1

== matlab function SiDLEngine/Deep Learning LSTM/MATLAB Function ==
  data: x input; y output; muX parameter; muY parameter; sigX parameter; sigY parameter; layer2InputWeights input; layer2RecurrentWeights input; layer2Bias input; layer3Weights input; layer3Bias input
function y = callLstmNet(x, muX, muY, sigX, sigY,layer2InputWeights,layer2RecurrentWeights,layer2Bias,layer3Weights,layer3Bias)
   y=autoblkssilstmeval(x,muX,muY,sigX,sigY,layer2InputWeights,layer2RecurrentWeights,layer2Bias,layer3Weights,layer3Bias);
end
